simulink model "import_data"  (R2022b)
settings: Solver=ode4  StartTime=0.0  StopTime=10.0  FixedStep=0.001  RelTol=1e-3
settings Model: Creator=craft  LastModifiedBy=craft

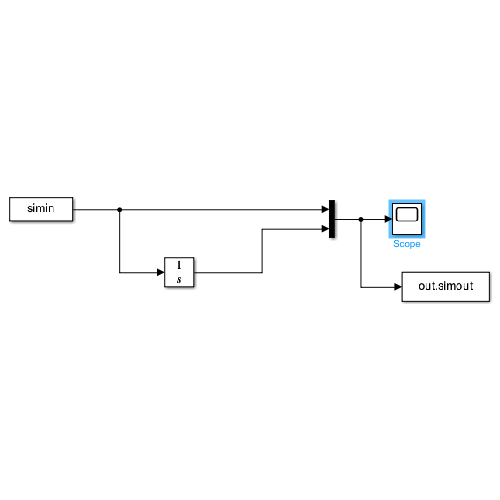
[thumbnail: Simulink's stored preview of the top-level diagram]
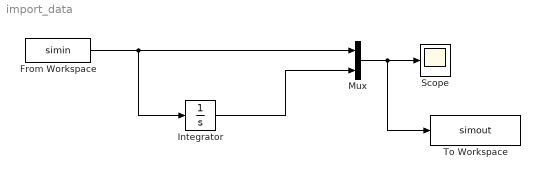
== system import_data ==
  From Workspace : FromWorkspace  VariableName=simin  OutputAfterFinalValue=Holding final value
  Integrator : Integrator
  Mux : Mux  Inputs=2
  Scope : Scope
  To Workspace : ToWorkspace  VariableName=simout  SaveFormat=Structure With Time  SampleTime=-1
  wires:
  From Workspace/1 -> Integrator/1, Mux/1
  Mux/1 -> To Workspace/1, Scope/1
  Integrator/1 -> Mux/2
